simulink model "L3_T1_linear"  (R2026a)
settings: Solver=ode23tb  StartTime=0  StopTime=40  MaxStep=0.002
settings Model: Creator=m  LastModifiedBy=m

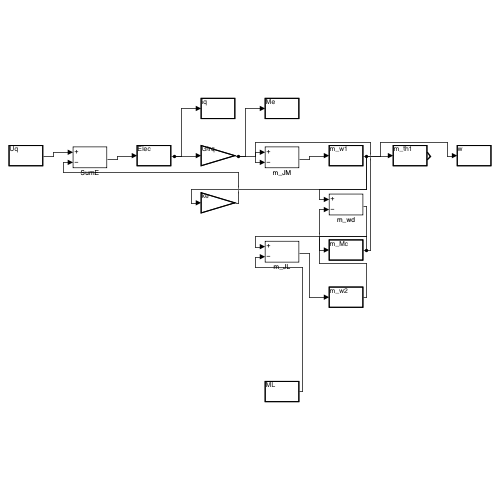
[thumbnail: Simulink's stored preview of the top-level diagram]
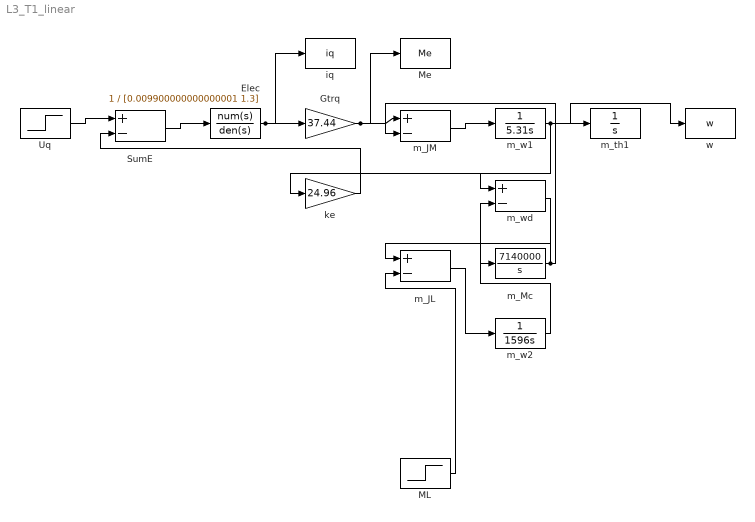
== system L3_T1_linear ==
  Elec : TransferFcn  Numerator=1  Denominator=[0.009900000000000001 1.3]
  Gtrq : Gain  Gain=37.44
  ML : Step  Time=20  FinalValue=100  SampleTime=0
  Me : ToWorkspace  VariableName=Me  SaveFormat=Structure With Time  SampleTime=-1
  SumE : Sum  Inputs=+-
  Uq : Step  Time=0  FinalValue=380.9113043478261  SampleTime=0
  iq : ToWorkspace  VariableName=iq  SaveFormat=Structure With Time  SampleTime=-1
  ke : Gain  Gain=24.96
  m_JL : Sum  Inputs=+-
  m_JM : Sum  Inputs=+-
  m_Mc : TransferFcn  Numerator=7140000  Denominator=[1 0]
  m_th1 : Integrator
  m_w1 : TransferFcn  Numerator=1  Denominator=[5.31 0]
  m_w2 : TransferFcn  Numerator=1  Denominator=[1596 0]
  m_wd : Sum  Inputs=+-
  w : ToWorkspace  VariableName=w  SaveFormat=Structure With Time  SampleTime=-1
  wires:
  m_JM/1 -> m_w1/1
  m_w1/1 -> m_wd/1, m_th1/1, ke/1, w/1
  m_w2/1 -> m_wd/2
  m_wd/1 -> m_Mc/1
  m_Mc/1 -> m_JM/2, m_JL/1
  m_JL/1 -> m_w2/1
  Uq/1 -> SumE/1
  ke/1 -> SumE/2
  SumE/1 -> Elec/1
  Elec/1 -> Gtrq/1, iq/1
  Gtrq/1 -> m_JM/1, Me/1
  ML/1 -> m_JL/2
